simulink model "SF028A_AssiHiFrq"  (R2013b)
settings: Solver=VariableStepDiscrete  StartTime=0.0  StopTime=10.0  RelTol=1e-3
values from neighbouring files (symbols this model uses):
  AssiHiFrqGainY = DataDict.Calibration    [SF028A_AssiHiFrq_DataDict.m]
  AssiHiFrqHpFilFrqY = DataDict.Calibration    [SF028A_AssiHiFrq_DataDict.m]
  AssiHiFrqTqWhlImbRejctnTqX = DataDict.Calibration    [SF028A_AssiHiFrq_DataDict.m]
  AssiHiFrqTqX = DataDict.Calibration    [SF028A_AssiHiFrq_DataDict.m]
  AssiHiFrqWhlImbRejctnGainY = DataDict.Calibration    [SF028A_AssiHiFrq_DataDict.m]
  AssiHiFrqWhlImbRejtcnBlndX = DataDict.Calibration    [SF028A_AssiHiFrq_DataDict.m]
  AssiHiFrqWhlImbRejtcnBlndY = DataDict.Calibration    [SF028A_AssiHiFrq_DataDict.m]
  SYSGLBPRM_MOTTQCMDHILIM_MOTNWTMTR_F32 = DataDict.Constant    [SF028A_AssiHiFrq_DataDict.m]
  SYSGLBPRM_MOTTQCMDLOLIM_MOTNWTMTR_F32 = DataDict.Constant    [SF028A_AssiHiFrq_DataDict.m]
  SysGlbPrmVehSpdBilnrSeln = DataDict.ImprtdCal    [SF028A_AssiHiFrq_DataDict.m]
undefined symbols (not defined in the file or in its folder): ARCHGLBPRM_2MILLISEC_SEC_F32, magnitude
libraries: simulink x6
Description:
  | This function provides a means of compensating for system inertia and road feedback.  It is
  |  tunable over both vehicle speed and handwheel torque to obtain the desired level of disurbance
  |  rejection under various operating conditions.  It passes handwheel torque through a high-pass
  |  filter and multiplies the resulting signal by a tunable gain factor.  The output is known as
  |  high-frequency assist and is simply added to the usual assist calculated elsewhere.
settings Model: Creator=lzz0tm  LastModifiedBy=HZZRQQ
settings Model: ModifiedHistory=|
  | 001
  | Initial release
  | K. Derry
  | 3-Nov-2011
  | n/a
  | 
  | 002
  | Use common vehicle speed table from SF-00
  | Reduce Torq tables from 32x16 to 13x12
  | Eliminate filter cutoff frequency WIR blending
  | Update to floating point high pass filter.
  | Changed filter cutoff required resolution from 0.005 Hz to 0.125 Hz.
  | Renamed 2-D cal tables from '...t..' to '..t2..' format.
  | Redefined display variables.
  | Eliminate Word doc.
  | K. Derry
  | 13-Mar-2013
  | ICR-4006
settings DataIOCC: SignalLoggingSaveFormat=ModelDataLogs  SaveOutput=off  DSMLogging=off  SaveTime=off
settings OptimizationCC: ExpressionDepthLimit=2147483647
settings DebuggingCC: FcnCallInpInsideContextMsg=UseLocalSettings  StateNameClashWarn=warning
settings GRTTargetCC: CombineOutputUpdateFcns=off  GRTInterface=on

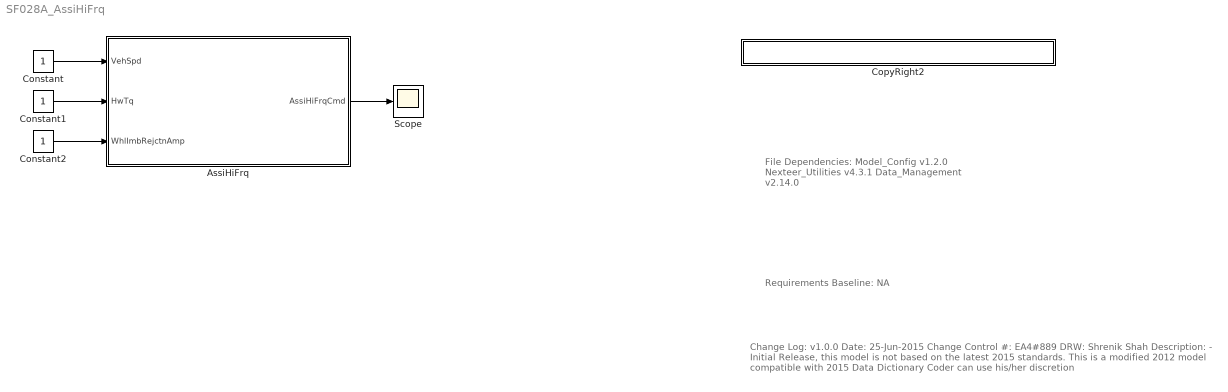
== system SF028A_AssiHiFrq ==
  note: File Dependencies:
      |
      | Model_Config v1.2.0
      | Nexteer_Utilities v4.3.1
      | Data_Management v2.14.0
  note: Requirements Baseline: NA
  note: Change Log:
      | v1.0.0
      | Date: 25-Jun-2015
      | Change Control #: EA4#889
      | DRW:  Shrenik Shah
      | Description:
      | - Initial Release, this model is not based on the latest 2015 standards.
      |   This is a modified 2012 model compatible with 2015 Data Dictionary
      |   Coder can use his/her discretion
  AssiHiFrq : Subsystem
  Constant : Constant
  Constant1 : Constant
  Constant2 : Constant
  CopyRight2 : Subsystem  Description=|  mask(Copyright Information){none=on}
      | Copyright info block.                                               
      |                                                                     
      | Place copyright information at the top of every subsystem in design.
      mask prompts: none "No parameters"
      mask help: Place copyright information at the top of every subsystem in design.
      mask Display:
      | NxtrConf = 'Nexteer Confidential';
      | 
      | sys = bdroot; %handle for the current model ("system")
      | first = get_param(sys,'Created');
      | if(isempty(first))
      |     first = datestr(now,'yyyy');
      | else
      |     first = first(end-3:end);  %year is last four digits
      | end
      | 
      | last = get_param(sys,'LastModifiedDate');
      | if isempty(last)
      |     last = datestr(now,'yyyy');
      | else
      |     last = last(end-3:end);
      | end
      | 
      | if strcmp(first,last)
      |     fprintf('%s -- Copyright %s Nexteer',NxtrConf,first)
      | else
      |     fprintf('%s -- %s%s- %s Nexteer',NxtrConf,char(169),first,last)
      | end
  Scope : Scope
  wires:
  Constant/1 -> AssiHiFrq/1(VehSpd)
  Constant1/1 -> AssiHiFrq/2(HwTq)
  Constant2/1 -> AssiHiFrq/3(WhlImbRejctnAmp)
  AssiHiFrq/1(AssiHiFrqCmd) -> Scope/1

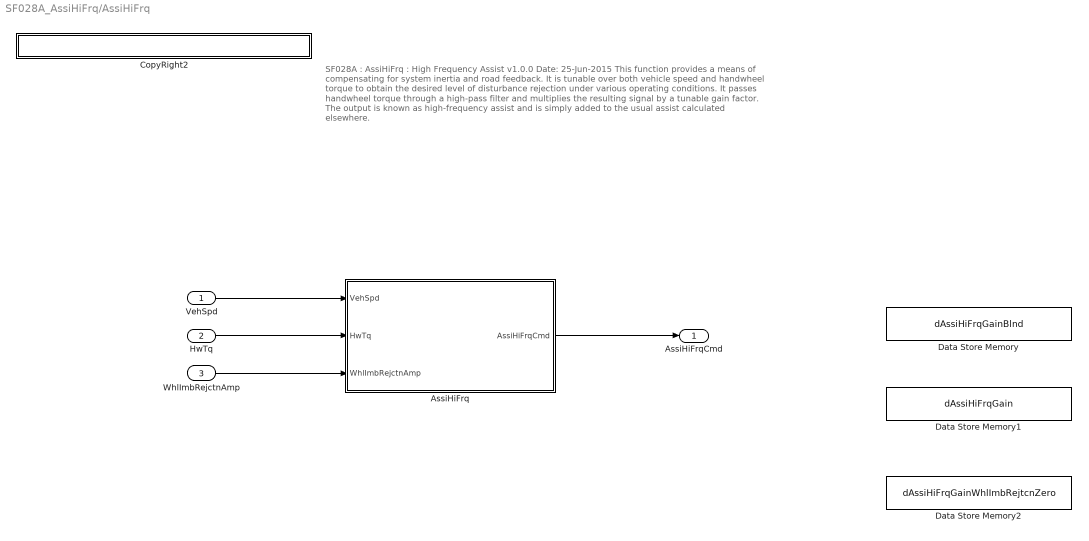
== system SF028A_AssiHiFrq/AssiHiFrq ==
  note: SF028A : AssiHiFrq : High Frequency Assist
      | v1.0.0
      | Date: 25-Jun-2015
      |
      |   This function provides a means of compensating for system inertia and
      |   road feedback. It is tunable over both vehicle speed and handwheel torque
      |   to obtain the desired level of disturbance rejection under various operating
      |   conditions. It passes handwheel torque through a high-pass filter and multiplies
      |   the resulting signal by a tunable gain factor. The output is known as high-frequency
      |   assist and is simply added to the usual assist calculated elsewhere.
  VehSpd : Inport
  HwTq : Inport  Port=2
  WhlImbRejctnAmp : Inport  Port=3
  AssiHiFrq : Subsystem
  CopyRight2 : Subsystem  Description=|  mask(Copyright Information){none=on}
      | Copyright info block.                                               
      |                                                                     
      | Place copyright information at the top of every subsystem in design.
      mask prompts: none "No parameters"
      mask help: Place copyright information at the top of every subsystem in design.
      mask Display:
      | NxtrConf = 'Nexteer Confidential';
      | 
      | sys = bdroot; %handle for the current model ("system")
      | first = get_param(sys,'Created');
      | if(isempty(first))
      |     first = datestr(now,'yyyy');
      | else
      |     first = first(end-3:end);  %year is last four digits
      | end
      | 
      | last = get_param(sys,'LastModifiedDate');
      | if isempty(last)
      |     last = datestr(now,'yyyy');
      | else
      |     last = last(end-3:end);
      | end
      | 
      | if strcmp(first,last)
      |     fprintf('%s -- Copyright %s Nexteer',NxtrConf,first)
      | else
      |     fprintf('%s -- %s%s- %s Nexteer',NxtrConf,char(169),first,last)
      | end
  Data Store Memory : DataStoreMemory  DataStoreName=dAssiHiFrqGainBlnd  ReadBeforeWriteMsg=warning  WriteAfterWriteMsg=warning  WriteAfterReadMsg=warning  StateMustResolveToSignalObject=on
  Data Store Memory1 : DataStoreMemory  DataStoreName=dAssiHiFrqGain  ReadBeforeWriteMsg=warning  WriteAfterWriteMsg=warning  WriteAfterReadMsg=warning  StateMustResolveToSignalObject=on
  Data Store Memory2 : DataStoreMemory  DataStoreName=dAssiHiFrqGainWhlImbRejtcnZero  ReadBeforeWriteMsg=warning  WriteAfterWriteMsg=warning  WriteAfterReadMsg=warning  StateMustResolveToSignalObject=on
  AssiHiFrqCmd : Outport
  wires:
  VehSpd/1 -> AssiHiFrq/1(VehSpd)
  HwTq/1 -> AssiHiFrq/2(HwTq)
  WhlImbRejctnAmp/1 -> AssiHiFrq/3(WhlImbRejctnAmp)
  AssiHiFrq/1(AssiHiFrqCmd) -> AssiHiFrqCmd/1

== system SF028A_AssiHiFrq/CopyRight2 ==

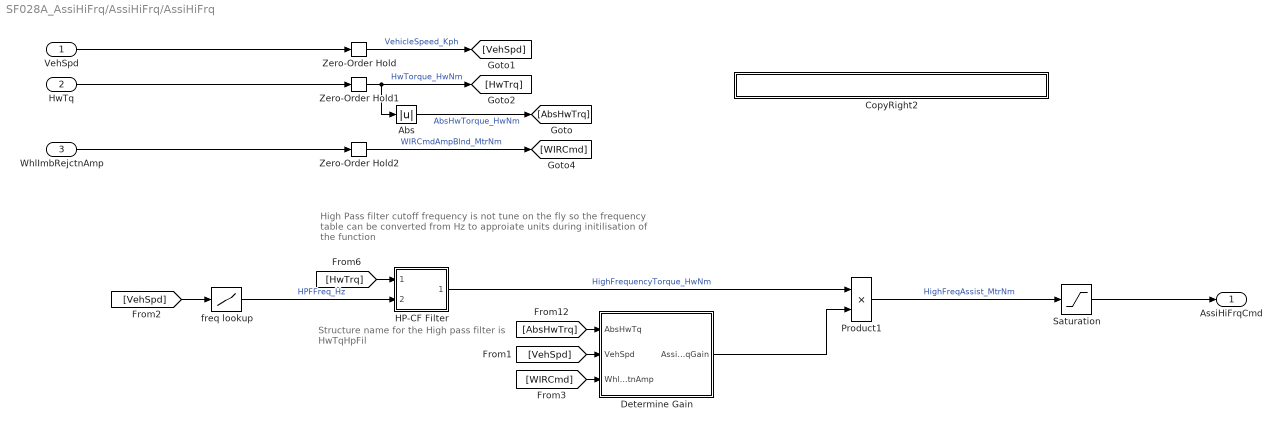
== system SF028A_AssiHiFrq/AssiHiFrq/AssiHiFrq ==
  note: Structure name for the High pass filter is
      | HwTqHpFil
  note: High Pass filter cutoff frequency is not tune on the fly
      | so the frequency table can be converted from Hz to approiate units
      | during initilisation of the function
  VehSpd : Inport
  HwTq : Inport  Port=2
  WhlImbRejctnAmp : Inport  Port=3
  Abs : Abs
  CopyRight2 : Subsystem  Description=|  mask(Copyright Information){none=on}
      | Copyright info block.                                               
      |                                                                     
      | Place copyright information at the top of every subsystem in design.
      mask prompts: none "No parameters"
      mask help: Place copyright information at the top of every subsystem in design.
      mask Display:
      | NxtrConf = 'Nexteer Confidential';
      | 
      | sys = bdroot; %handle for the current model ("system")
      | first = get_param(sys,'Created');
      | if(isempty(first))
      |     first = datestr(now,'yyyy');
      | else
      |     first = first(end-3:end);  %year is last four digits
      | end
      | 
      | last = get_param(sys,'LastModifiedDate');
      | if isempty(last)
      |     last = datestr(now,'yyyy');
      | else
      |     last = last(end-3:end);
      | end
      | 
      | if strcmp(first,last)
      |     fprintf('%s -- Copyright %s Nexteer',NxtrConf,first)
      | else
      |     fprintf('%s -- %s%s- %s Nexteer',NxtrConf,char(169),first,last)
      | end
  Determine Gain : Subsystem
  HP-CF Filter : Subsystem  mask(HP-CF Filter){Ts_sec=ARCHGLBPRM_2MILLISEC_SEC_F32, LP_IC=0}
      mask prompts: Ts_sec "Function Time Step (seconds)"; LP_IC "Input Signal Initial Condition (Engineering Units)"
      mask help:
      | version:  Mar 27, 2013
      |
      | REVISIONS
      |   Mar 05, 2012.  Date created.
      |   Mar 16, 2012.  corr_factor changed.  (see mask initialization).
      |   May 22, 2012.  Added cutoff freq as inport.
      |   Mar 27, 2013.  Updated LPF block and fixed error.  LPF was using hardcoded parameters.
      mask init:
      | g = 2*pi*Ts_sec;
      mask Display:
      | port_label('input',1,'y')
      | port_label('input',2,'Hz')
      | 
      | %a = [2:0.1:5.2]';
      | %b = sin(2*a);
      | %c = 0.5*sin(25*a);
      | %d = b+c;
      | %e = vertcat(d, c);
      | %plot(e);
      | 
      | disp 'HPF'
  Product1 : Product  OutDataTypeStr=float('double')  SaturateOnIntegerOverflow=on  InputSameDT=on
  Saturation : Saturate  UpperLimit=SYSGLBPRM_MOTTQCMDHILIM_MOTNWTMTR_F32  LowerLimit=SYSGLBPRM_MOTTQCMDLOLIM_MOTNWTMTR_F32
  Zero-Order Hold : ZeroOrderHold  SampleTime=ARCHGLBPRM_2MILLISEC_SEC_F32
  Zero-Order Hold1 : ZeroOrderHold  SampleTime=ARCHGLBPRM_2MILLISEC_SEC_F32
  Zero-Order Hold2 : ZeroOrderHold  SampleTime=ARCHGLBPRM_2MILLISEC_SEC_F32
  freq lookup : Lookup  InputValues=SysGlbPrmVehSpdBilnrSeln  Table=AssiHiFrqHpFilFrqY  LookUpMeth=Interpolation-Use End Values  SaturateOnIntegerOverflow=on
      settings: AttributesFormatString=%<InputValues>\n%<Table>
  AssiHiFrqCmd : Outport
  wires:
  Product1/1 -> Saturation/1  "HighFreqAssist_MtrNm"
  VehSpd/1 -> Zero-Order Hold/1
  HwTq/1 -> Zero-Order Hold1/1
  Zero-Order Hold/1 -> [VehSpd]  "VehicleSpeed_Kph"
  Zero-Order Hold1/1 -> [HwTrq], Abs/1  "HwTorque_HwNm"
  Abs/1 -> [AbsHwTrq]  "AbsHwTorque_HwNm"
  WhlImbRejctnAmp/1 -> Zero-Order Hold2/1
  Zero-Order Hold2/1 -> [WIRCmd]  "WIRCmdAmpBlnd_MtrNm"
  HP-CF Filter/1(Output) -> Product1/1  "HighFrequencyTorque_HwNm"
  Determine Gain/1(AssiHiFrqGain) -> Product1/2
  [VehSpd] -> freq lookup/1
  [AbsHwTrq] -> Determine Gain/1(AbsHwTq)
  [VehSpd] -> Determine Gain/2(VehSpd)
  [WIRCmd] -> Determine Gain/3(WhlImbRejctnAmp)
  [HwTrq] -> HP-CF Filter/1(Input)
  freq lookup/1 -> HP-CF Filter/2(KnHz)  "HPFFreq_Hz"
  Saturation/1 -> AssiHiFrqCmd/1

== system SF028A_AssiHiFrq/AssiHiFrq/CopyRight2 ==

== system SF028A_AssiHiFrq/AssiHiFrq/AssiHiFrq/CopyRight2 ==

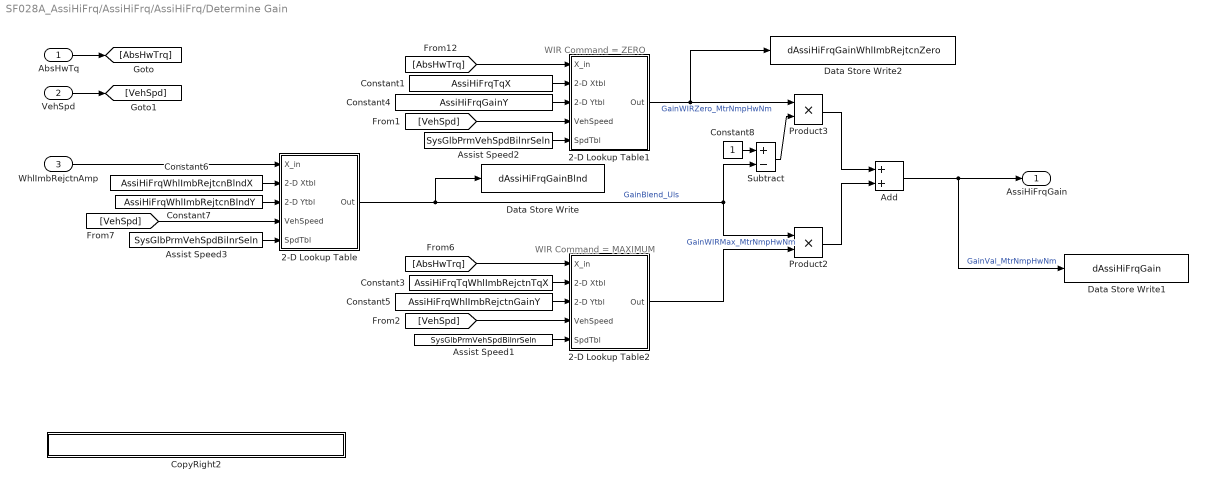
== system SF028A_AssiHiFrq/AssiHiFrq/AssiHiFrq/Determine Gain ==
  note: WIR Command = ZERO
  note: WIR Command = MAXIMUM
  AbsHwTq : Inport
  VehSpd : Inport  Port=2
  WhlImbRejctnAmp : Inport  Port=3
  2-D Lookup Table : Subsystem  mask(2-D Lookup Table){}
      mask help: version: Apr 19, 2012
  2-D Lookup Table1 : Subsystem  mask(2-D Lookup Table){}
      mask help: version: Apr 19, 2012
  2-D Lookup Table2 : Subsystem  mask(2-D Lookup Table){}
      mask help: version: Apr 19, 2012
  Add : Sum
  Assist Speed1 : Constant  Value=SysGlbPrmVehSpdBilnrSeln
  Assist Speed2 : Constant  Value=SysGlbPrmVehSpdBilnrSeln
  Assist Speed3 : Constant  Value=SysGlbPrmVehSpdBilnrSeln
  Constant1 : Constant  Value=AssiHiFrqTqX
  Constant3 : Constant  Value=AssiHiFrqTqWhlImbRejctnTqX
  Constant4 : Constant  Value=AssiHiFrqGainY
  Constant5 : Constant  Value=AssiHiFrqWhlImbRejctnGainY
  Constant6 : Constant  Value=AssiHiFrqWhlImbRejtcnBlndX
  Constant7 : Constant  Value=AssiHiFrqWhlImbRejtcnBlndY
  Constant8 : Constant
  CopyRight2 : Subsystem  Description=|  mask(Copyright Information){none=on}
      | Copyright info block.                                               
      |                                                                     
      | Place copyright information at the top of every subsystem in design.
      mask prompts: none "No parameters"
      mask help: Place copyright information at the top of every subsystem in design.
      mask Display:
      | NxtrConf = 'Nexteer Confidential';
      | 
      | sys = bdroot; %handle for the current model ("system")
      | first = get_param(sys,'Created');
      | if(isempty(first))
      |     first = datestr(now,'yyyy');
      | else
      |     first = first(end-3:end);  %year is last four digits
      | end
      | 
      | last = get_param(sys,'LastModifiedDate');
      | if isempty(last)
      |     last = datestr(now,'yyyy');
      | else
      |     last = last(end-3:end);
      | end
      | 
      | if strcmp(first,last)
      |     fprintf('%s -- Copyright %s Nexteer',NxtrConf,first)
      | else
      |     fprintf('%s -- %s%s- %s Nexteer',NxtrConf,char(169),first,last)
      | end
  Data Store Write : DataStoreWrite  DataStoreName=dAssiHiFrqGainBlnd
  Data Store Write1 : DataStoreWrite  DataStoreName=dAssiHiFrqGain
  Data Store Write2 : DataStoreWrite  DataStoreName=dAssiHiFrqGainWhlImbRejtcnZero
  Product2 : Product  RndMeth=Zero
  Product3 : Product  RndMeth=Zero
  Subtract : Sum  Inputs=+-
  AssiHiFrqGain : Outport
  wires:
  [AbsHwTrq] -> 2-D Lookup Table1/1(X_in)
  Assist Speed2/1 -> 2-D Lookup Table1/5(SpdTbl)
  Constant1/1 -> 2-D Lookup Table1/2(2-D Xtbl)
  Constant4/1 -> 2-D Lookup Table1/3(2-D Ytbl)
  [VehSpd] -> 2-D Lookup Table1/4(VehSpeed)
  [AbsHwTrq] -> 2-D Lookup Table2/1(X_in)
  Assist Speed1/1 -> 2-D Lookup Table2/5(SpdTbl)
  Constant5/1 -> 2-D Lookup Table2/3(2-D Ytbl)
  [VehSpd] -> 2-D Lookup Table2/4(VehSpeed)
  Assist Speed3/1 -> 2-D Lookup Table/5(SpdTbl)
  Constant6/1 -> 2-D Lookup Table/2(2-D Xtbl)
  Constant7/1 -> 2-D Lookup Table/3(2-D Ytbl)
  [VehSpd] -> 2-D Lookup Table/4(VehSpeed)
  2-D Lookup Table/1(Out) -> Data Store Write/1, Product2/1, Subtract/2  "GainBlend_Uls"
  2-D Lookup Table2/1(Out) -> Product2/2  "GainWIRMax_MtrNmpHwNm"
  Constant8/1 -> Subtract/1
  2-D Lookup Table1/1(Out) -> Data Store Write2/1, Product3/1  "GainWIRZero_MtrNmpHwNm"
  Subtract/1 -> Product3/2
  Product3/1 -> Add/1
  Product2/1 -> Add/2
  Constant3/1 -> 2-D Lookup Table2/2(2-D Xtbl)
  Add/1 -> Data Store Write1/1, AssiHiFrqGain/1  "GainVal_MtrNmpHwNm"
  VehSpd/1 -> [VehSpd]
  AbsHwTq/1 -> [AbsHwTrq]
  WhlImbRejctnAmp/1 -> 2-D Lookup Table/1(X_in)

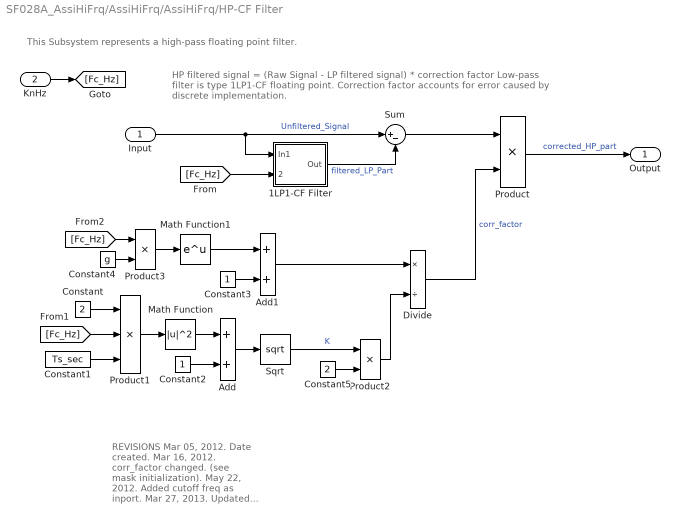
== system SF028A_AssiHiFrq/AssiHiFrq/AssiHiFrq/HP-CF Filter ==
  note: HP filtered signal = (Raw Signal - LP filtered signal) * correction factor
      |
      | Low-pass filter is type 1LP1-CF floating point.
      | Correction factor accounts for error caused by discrete implementation.
  note: REVISIONS
      |   Mar 05, 2012.  Date created.
      |   Mar 16, 2012.  corr_factor changed.  (see mask initialization).
      |   May 22, 2012.  Added cutoff freq as inport.
      |   Mar 27, 2013.  Updated LPF block and fixed error.  LPF was using hardcoded parameters.
  note: This Subsystem represents a high-pass floating point filter.
  Input : Inport
  KnHz : Inport  Port=2
  " 1LP1-CF Filter " : Subsystem  mask(1LP1-CF Filter){Ts=Ts_sec, IC=LP_IC}
      mask prompts: Ts "Function Time Step (seconds)"; IC "Initial Condition (Enineering Units)"
      mask help: version: Mar 11, 2013
      settings: AttributesFormatString="time:  %<Ts>\\nI.C.:   %<IC>"
      mask Display:
      | port_label('input',1,'y')
      | port_label('input',2,'Hz')
      | 
      | %a = [2:0.1:5.2]';
      | %b = sin(2*a);
      | %c = 0.7*sin(25*a);
      | %d = b+c;
      | %e = vertcat(d, b);
      | %plot(e);
      | 
      | disp 'LPF'
  Add : Sum
  Add1 : Sum
  Constant : Constant  Value=2
  Constant1 : Constant  Value=Ts_sec
  Constant2 : Constant
  Constant3 : Constant
  Constant4 : Constant  Value=g
  Constant5 : Constant  Value=2
  Divide : Product  Inputs=*/
  Math Function : Math  Operator=magnitude^2  SaturateOnIntegerOverflow=on
  Math Function1 : Math  SaturateOnIntegerOverflow=on
  Product : Product  RndMeth=Zero
  Product1 : Product  Inputs=3  RndMeth=Zero
  Product2 : Product  RndMeth=Zero
  Product3 : Product  RndMeth=Zero
  Sqrt : Sqrt  SaturateOnIntegerOverflow=on
  Sum : Sum  Inputs=|+-
  Output : Outport
  wires:
  [Fc_Hz] -> " 1LP1-CF Filter "/2(KnHz)
  Input/1 -> Sum/1, " 1LP1-CF Filter "/1(In1)  "Unfiltered_Signal"
  " 1LP1-CF Filter "/1(Out) -> Sum/2  "filtered_LP_Part"
  Sum/1 -> Product/1
  Product/1 -> Output/1  "corrected_HP_part"
  Constant/1 -> Product1/1
  KnHz/1 -> [Fc_Hz]
  Product1/1 -> Math Function/1
  Math Function/1 -> Add/1
  Constant2/1 -> Add/2
  Add/1 -> Sqrt/1
  Constant3/1 -> Add1/2
  Math Function1/1 -> Add1/1
  Sqrt/1 -> Product2/1  "K"
  Constant5/1 -> Product2/2
  Product3/1 -> Math Function1/1
  [Fc_Hz] -> Product3/1
  Constant4/1 -> Product3/2
  [Fc_Hz] -> Product1/2
  Constant1/1 -> Product1/3
  Add1/1 -> Divide/1
  Product2/1 -> Divide/2
  Divide/1 -> Product/2  "corr_factor"

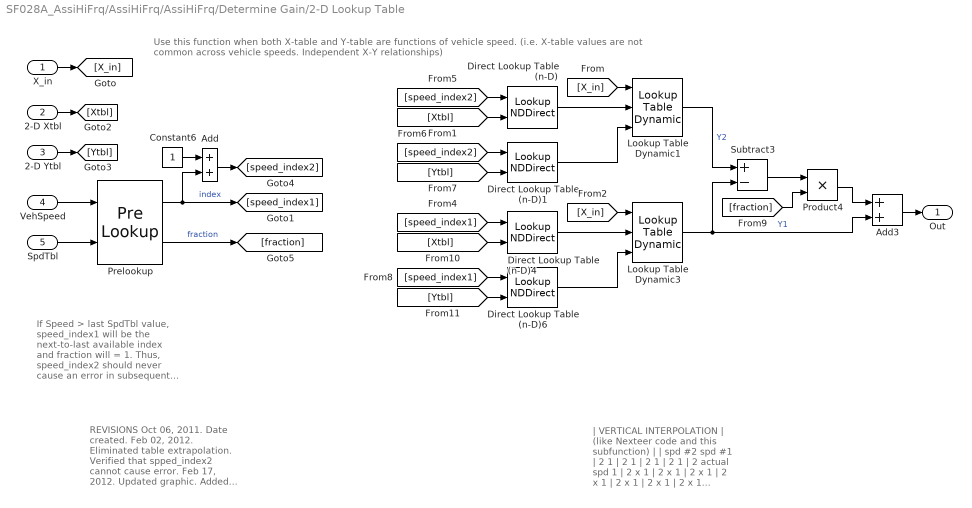
== system SF028A_AssiHiFrq/AssiHiFrq/AssiHiFrq/Determine Gain/2-D Lookup Table ==
  note: REVISIONS
      |   Oct 06, 2011.  Date created.
      |   Feb 02, 2012.  Eliminated table extrapolation.  Verified that spped_index2 cannot cause error.
      |   Feb 17, 2012.  Updated graphic.  Added this revision block.
      |   Apr  19, 2012.  Renamed Speed to VehSpeed for clarity.
  note: |         VERTICAL INTERPOLATION
      | |                    (like Nexteer code and this subfunction)
      | |
      | |                                        spd #2                    spd #1
      | |                                           2                             1
      | |                                         2                            1
      | |                                       2                           1
      | |                                    2                           1
      | |                                 2     actual spd      1
      | |                              2            x             1
      | |                           2            x            1
      | |                        2            x            1
      | |                    2            x             1
      | |                 2           x             1
      | |            2        x                 1
      | |     2         x                  1
      | |2_x_____________1_____________________________
  note: Use this function when both X-table and Y-table are functions of vehicle speed.
      | (i.e. X-table values are not common across vehicle speeds.  Independent X-Y relationships)
  note: If Speed > last SpdTbl value, speed_index1 will be the
      | next-to-last available index and fraction will = 1.  Thus,
      | speed_index2 should never cause an error in subsequent
      | lookup tables.
  X_in : Inport
  2-D Xtbl : Inport  Port=2
  2-D Ytbl : Inport  Port=3
  VehSpeed : Inport  Port=4
  SpdTbl : Inport  Port=5
  Add : Sum
  Add3 : Sum
  Constant6 : Constant
  Direct Lookup Table (n-D){,1,4,6} (4 alike) : LookupNDDirect  InputsSelectThisObjectFromTable=Column  TableIsInput=on
  Lookup Table Dynamic1 : simulink/Lookup Tables/Lookup Table Dynamic  LookUpMeth=Interpolation-Use End Values  OutDataTypeStr=fixdt('double')  OutputDataTypeScalingMode=Specify via dialog  OutDataType=fixdt('double')  OutScaling=2^-10  DoSatur=off
  Lookup Table Dynamic3 : simulink/Lookup Tables/Lookup Table Dynamic  LookUpMeth=Interpolation-Use End Values  OutDataTypeStr=fixdt('double')  OutputDataTypeScalingMode=Specify via dialog  OutDataType=fixdt('double')  OutScaling=2^-10  DoSatur=off
  Prelookup : PreLookup  BreakpointsDataSource=Input port  BreakpointsData=[10:10:110]
      settings: InputPortMap=u0,p1
  Product4 : Product  RndMeth=Zero
  Subtract3 : Sum  Inputs=+-
  Out : Outport
  wires:
  Add3/1 -> Out/1
  SpdTbl/1 -> Prelookup/2
  Prelookup/2 -> [fraction]  "fraction"
  Add/1 -> [speed_index2]
  Prelookup/1 -> Add/2, [speed_index1]  "index"
  Constant6/1 -> Add/1
  VehSpeed/1 -> Prelookup/1
  X_in/1 -> [X_in]
  2-D Ytbl/1 -> [Ytbl]
  2-D Xtbl/1 -> [Xtbl]
  [fraction] -> Product4/2
  Lookup Table Dynamic3/1 -> Add3/2, Subtract3/2  "Y1"
  [speed_index1] -> Direct Lookup Table (n-D)6/1
  [speed_index1] -> Direct Lookup Table (n-D)4/1
  [speed_index2] -> Direct Lookup Table (n-D)1/1
  [speed_index2] -> Direct Lookup Table (n-D)/1
  [X_in] -> Lookup Table Dynamic3/1
  Direct Lookup Table (n-D)6/1 -> Lookup Table Dynamic3/3
  Direct Lookup Table (n-D)4/1 -> Lookup Table Dynamic3/2
  [Ytbl] -> Direct Lookup Table (n-D)6/2
  [Xtbl] -> Direct Lookup Table (n-D)4/2
  [X_in] -> Lookup Table Dynamic1/1
  Direct Lookup Table (n-D)1/1 -> Lookup Table Dynamic1/3
  Direct Lookup Table (n-D)/1 -> Lookup Table Dynamic1/2
  [Ytbl] -> Direct Lookup Table (n-D)1/2
  [Xtbl] -> Direct Lookup Table (n-D)/2
  Product4/1 -> Add3/1
  Subtract3/1 -> Product4/1
  Lookup Table Dynamic1/1 -> Subtract3/1  "Y2"

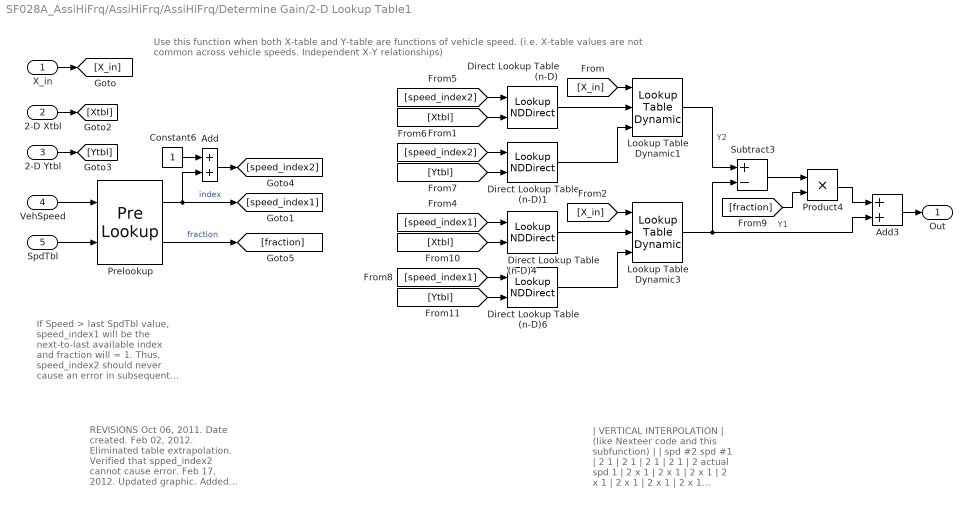
== system SF028A_AssiHiFrq/AssiHiFrq/AssiHiFrq/Determine Gain/2-D Lookup Table1 ==
  note: If Speed > last SpdTbl value, speed_index1 will be the
      | next-to-last available index and fraction will = 1.  Thus,
      | speed_index2 should never cause an error in subsequent
      | lookup tables.
  note: Use this function when both X-table and Y-table are functions of vehicle speed.
      | (i.e. X-table values are not common across vehicle speeds.  Independent X-Y relationships)
  note: |         VERTICAL INTERPOLATION
      | |                    (like Nexteer code and this subfunction)
      | |
      | |                                        spd #2                    spd #1
      | |                                           2                             1
      | |                                         2                            1
      | |                                       2                           1
      | |                                    2                           1
      | |                                 2     actual spd      1
      | |                              2            x             1
      | |                           2            x            1
      | |                        2            x            1
      | |                    2            x             1
      | |                 2           x             1
      | |            2        x                 1
      | |     2         x                  1
      | |2_x_____________1_____________________________
  note: REVISIONS
      |   Oct 06, 2011.  Date created.
      |   Feb 02, 2012.  Eliminated table extrapolation.  Verified that spped_index2 cannot cause error.
      |   Feb 17, 2012.  Updated graphic.  Added this revision block.
      |   Apr  19, 2012.  Renamed Speed to VehSpeed for clarity.
  X_in : Inport
  2-D Xtbl : Inport  Port=2
  2-D Ytbl : Inport  Port=3
  VehSpeed : Inport  Port=4
  SpdTbl : Inport  Port=5
  Add : Sum
  Add3 : Sum
  Constant6 : Constant
  Direct Lookup Table (n-D){,1,4,6} (4 alike) : LookupNDDirect  InputsSelectThisObjectFromTable=Column  TableIsInput=on
  Lookup Table Dynamic1 : simulink/Lookup Tables/Lookup Table Dynamic  LookUpMeth=Interpolation-Use End Values  OutDataTypeStr=fixdt('double')  OutputDataTypeScalingMode=Specify via dialog  OutDataType=fixdt('double')  OutScaling=2^-10  DoSatur=off
  Lookup Table Dynamic3 : simulink/Lookup Tables/Lookup Table Dynamic  LookUpMeth=Interpolation-Use End Values  OutDataTypeStr=fixdt('double')  OutputDataTypeScalingMode=Specify via dialog  OutDataType=fixdt('double')  OutScaling=2^-10  DoSatur=off
  Prelookup : PreLookup  BreakpointsDataSource=Input port  BreakpointsData=[10:10:110]
      settings: InputPortMap=u0,p1
  Product4 : Product  RndMeth=Zero
  Subtract3 : Sum  Inputs=+-
  Out : Outport
  wires:
  Lookup Table Dynamic1/1 -> Subtract3/1  "Y2"
  Subtract3/1 -> Product4/1
  Product4/1 -> Add3/1
  [Xtbl] -> Direct Lookup Table (n-D)/2
  [Ytbl] -> Direct Lookup Table (n-D)1/2
  Direct Lookup Table (n-D)/1 -> Lookup Table Dynamic1/2
  Direct Lookup Table (n-D)1/1 -> Lookup Table Dynamic1/3
  [X_in] -> Lookup Table Dynamic1/1
  [Xtbl] -> Direct Lookup Table (n-D)4/2
  [Ytbl] -> Direct Lookup Table (n-D)6/2
  Direct Lookup Table (n-D)4/1 -> Lookup Table Dynamic3/2
  Direct Lookup Table (n-D)6/1 -> Lookup Table Dynamic3/3
  [X_in] -> Lookup Table Dynamic3/1
  [speed_index2] -> Direct Lookup Table (n-D)/1
  [speed_index2] -> Direct Lookup Table (n-D)1/1
  [speed_index1] -> Direct Lookup Table (n-D)4/1
  [speed_index1] -> Direct Lookup Table (n-D)6/1
  Lookup Table Dynamic3/1 -> Subtract3/2, Add3/2  "Y1"
  [fraction] -> Product4/2
  2-D Xtbl/1 -> [Xtbl]
  2-D Ytbl/1 -> [Ytbl]
  X_in/1 -> [X_in]
  VehSpeed/1 -> Prelookup/1
  Constant6/1 -> Add/1
  Prelookup/1 -> [speed_index1], Add/2  "index"
  Add/1 -> [speed_index2]
  Prelookup/2 -> [fraction]  "fraction"
  SpdTbl/1 -> Prelookup/2
  Add3/1 -> Out/1

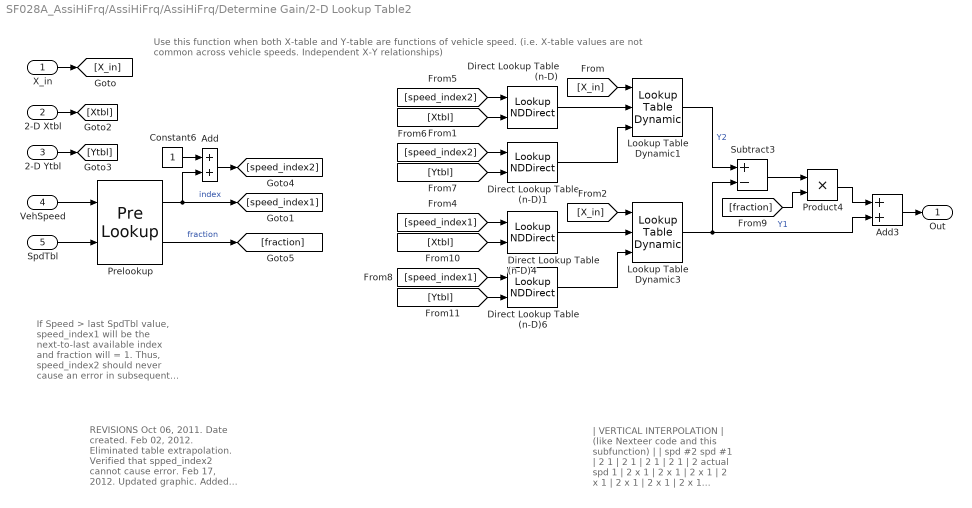
== system SF028A_AssiHiFrq/AssiHiFrq/AssiHiFrq/Determine Gain/2-D Lookup Table2 ==
  note: REVISIONS
      |   Oct 06, 2011.  Date created.
      |   Feb 02, 2012.  Eliminated table extrapolation.  Verified that spped_index2 cannot cause error.
      |   Feb 17, 2012.  Updated graphic.  Added this revision block.
      |   Apr  19, 2012.  Renamed Speed to VehSpeed for clarity.
  note: |         VERTICAL INTERPOLATION
      | |                    (like Nexteer code and this subfunction)
      | |
      | |                                        spd #2                    spd #1
      | |                                           2                             1
      | |                                         2                            1
      | |                                       2                           1
      | |                                    2                           1
      | |                                 2     actual spd      1
      | |                              2            x             1
      | |                           2            x            1
      | |                        2            x            1
      | |                    2            x             1
      | |                 2           x             1
      | |            2        x                 1
      | |     2         x                  1
      | |2_x_____________1_____________________________
  note: Use this function when both X-table and Y-table are functions of vehicle speed.
      | (i.e. X-table values are not common across vehicle speeds.  Independent X-Y relationships)
  note: If Speed > last SpdTbl value, speed_index1 will be the
      | next-to-last available index and fraction will = 1.  Thus,
      | speed_index2 should never cause an error in subsequent
      | lookup tables.
  X_in : Inport
  2-D Xtbl : Inport  Port=2
  2-D Ytbl : Inport  Port=3
  VehSpeed : Inport  Port=4
  SpdTbl : Inport  Port=5
  Add : Sum
  Add3 : Sum
  Constant6 : Constant
  Direct Lookup Table (n-D){,1,4,6} (4 alike) : LookupNDDirect  InputsSelectThisObjectFromTable=Column  TableIsInput=on
  Lookup Table Dynamic1 : simulink/Lookup Tables/Lookup Table Dynamic  LookUpMeth=Interpolation-Use End Values  OutDataTypeStr=fixdt('double')  OutputDataTypeScalingMode=Specify via dialog  OutDataType=fixdt('double')  OutScaling=2^-10  DoSatur=off
  Lookup Table Dynamic3 : simulink/Lookup Tables/Lookup Table Dynamic  LookUpMeth=Interpolation-Use End Values  OutDataTypeStr=fixdt('double')  OutputDataTypeScalingMode=Specify via dialog  OutDataType=fixdt('double')  OutScaling=2^-10  DoSatur=off
  Prelookup : PreLookup  BreakpointsDataSource=Input port  BreakpointsData=[10:10:110]
      settings: InputPortMap=u0,p1
  Product4 : Product  RndMeth=Zero
  Subtract3 : Sum  Inputs=+-
  Out : Outport
  wires:
  Add3/1 -> Out/1
  SpdTbl/1 -> Prelookup/2
  Prelookup/2 -> [fraction]  "fraction"
  Add/1 -> [speed_index2]
  Prelookup/1 -> Add/2, [speed_index1]  "index"
  Constant6/1 -> Add/1
  VehSpeed/1 -> Prelookup/1
  X_in/1 -> [X_in]
  2-D Ytbl/1 -> [Ytbl]
  2-D Xtbl/1 -> [Xtbl]
  [fraction] -> Product4/2
  Lookup Table Dynamic3/1 -> Add3/2, Subtract3/2  "Y1"
  [speed_index1] -> Direct Lookup Table (n-D)6/1
  [speed_index1] -> Direct Lookup Table (n-D)4/1
  [speed_index2] -> Direct Lookup Table (n-D)1/1
  [speed_index2] -> Direct Lookup Table (n-D)/1
  [X_in] -> Lookup Table Dynamic3/1
  Direct Lookup Table (n-D)6/1 -> Lookup Table Dynamic3/3
  Direct Lookup Table (n-D)4/1 -> Lookup Table Dynamic3/2
  [Ytbl] -> Direct Lookup Table (n-D)6/2
  [Xtbl] -> Direct Lookup Table (n-D)4/2
  [X_in] -> Lookup Table Dynamic1/1
  Direct Lookup Table (n-D)1/1 -> Lookup Table Dynamic1/3
  Direct Lookup Table (n-D)/1 -> Lookup Table Dynamic1/2
  [Ytbl] -> Direct Lookup Table (n-D)1/2
  [Xtbl] -> Direct Lookup Table (n-D)/2
  Product4/1 -> Add3/1
  Subtract3/1 -> Product4/1
  Lookup Table Dynamic1/1 -> Subtract3/1  "Y2"

== system SF028A_AssiHiFrq/AssiHiFrq/AssiHiFrq/Determine Gain/CopyRight2 ==

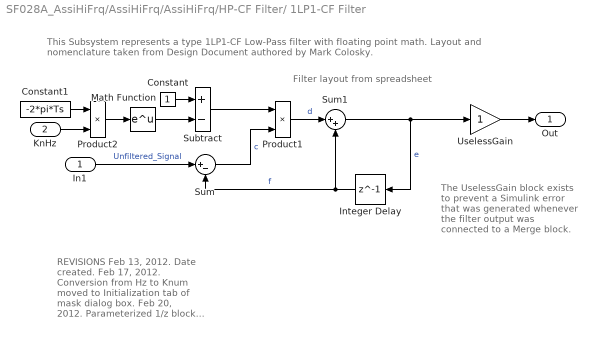
== system SF028A_AssiHiFrq/AssiHiFrq/AssiHiFrq/HP-CF Filter/ 1LP1-CF Filter  ==
  note: The UselessGain block exists to prevent
      | a Simulink error that was generated whenever
      | the filter output was connected to a Merge block.
  note: REVISIONS
      |   Feb 13, 2012.  Date created.
      |   Feb 17, 2012.  Conversion from Hz to Knum moved to Initialization tab of mask dialog box.
      |   Feb 20, 2012.  Parameterized 1/z block Initial Condition instead of hard-coded = 0.
      |   May 22, 2012.  Added external cutoff frequency signal.
      |   Mar 11, 2013.  Added UselessGain block for error prevention.
  note: This Subsystem represents a type 1LP1-CF Low-Pass filter with floating point math.
      | Layout and nomenclature taken from Design Document authored by Mark Colosky.
  note: Filter layout from spreadsheet
  In1 : Inport
  KnHz : Inport  Port=2
  Constant : Constant
  Constant1 : Constant  Value=-2*pi*Ts
  Integer Delay : Delay  DelayLength=1  InitialCondition=IC  SampleTime=Ts
  Math Function : Math  SaturateOnIntegerOverflow=on
  Product1 : Product  RndMeth=Zero
  Product2 : Product  RndMeth=Zero
  Subtract : Sum  Inputs=+-
  Sum : Sum  Inputs=|+-
  Sum1 : Sum  Inputs=|++
  UselessGain : Gain
  Out : Outport
  wires:
  UselessGain/1 -> Out/1
  Sum/1 -> Product1/2  "c"
  Product1/1 -> Sum1/1  "d"
  Integer Delay/1 -> Sum1/2, Sum/2  "f"
  In1/1 -> Sum/1  "Unfiltered_Signal"
  Sum1/1 -> UselessGain/1, Integer Delay/1  "e"
  Constant/1 -> Subtract/1
  Math Function/1 -> Subtract/2
  Constant1/1 -> Product2/1
  KnHz/1 -> Product2/2
  Product2/1 -> Math Function/1
  Subtract/1 -> Product1/1
